simulink model "PRBS_Para_CCPIDSim"  (R2015a)
settings: Solver=ode5  StartTime=0.0  StopTime=10  FixedStep=sim_stepSize
undefined symbols (not defined in the file or in its folder): sim_ccTarget, sim_PIDdGain, sim_PIDiGain, sim_PIDnoise, sim_PIDpGain, sim_PIDsample, sim_Qgain, sim_tracerMax, sim_zoneVolGain
libraries: simulink x8
settings Model: Creator=David  LastModifiedBy=davidveitch
settings SolverCC: NumberNewtonIterations=4  MaxConsecutiveMinStep=auto
settings DataIOCC: LimitDataPoints=off  SaveOutput=off  SignalLogging=off  DSMLogging=off  SaveTime=off  TimeSaveName=d_toutPRBS  OutputSaveName=Conc
settings OptimizationCC: ExpressionDepthLimit=2147483647  SimCompilerOptimization=on
settings DebuggingCC: UnderspecifiedInitializationDetection=Classic  MergeDetectMultiDrivingBlocksExec=none  SolverPrmCheckMsg=warning  MultiTaskRateTransMsg=warning  StateNameClashWarn=warning
settings ModelReferenceCC: UpdateModelReferenceTargets=IfOutOfDate
settings SFSimCC: SFSimEcho=off

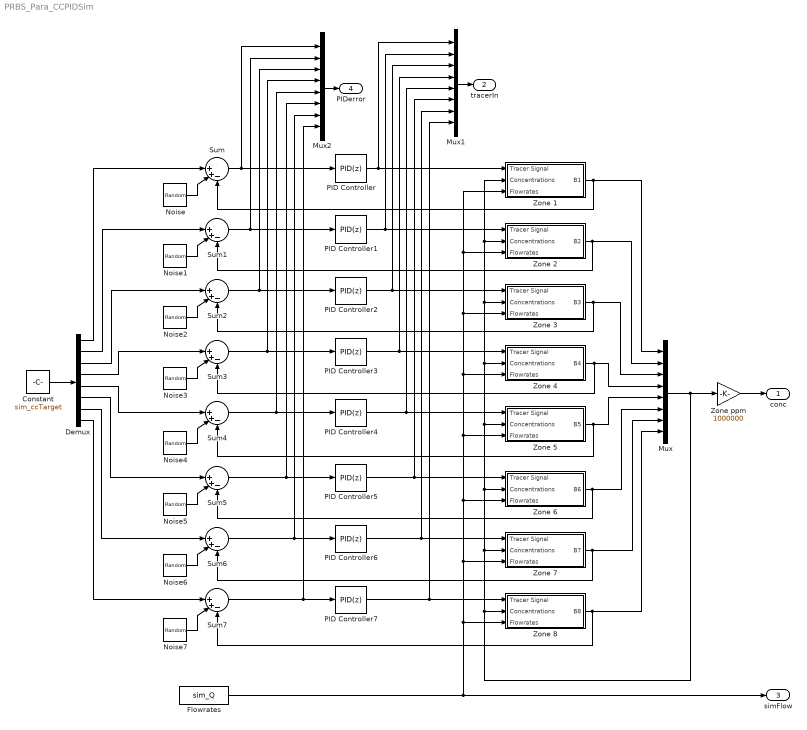
== system PRBS_Para_CCPIDSim ==
  Constant : Constant  Value=sim_ccTarget
  Demux : Demux  Outputs=8
  Flowrates : FromWorkspace  VariableName=sim_Q  SampleTime=0  OutputAfterFinalValue=Holding final value
  Mux : Mux  Inputs=8
  Mux1 : Mux  Inputs=8
  Mux2 : Mux  Inputs=8
  Noise : RandomNumber  Variance=sim_PIDnoise  Seed=100  SampleTime=sim_PIDsample
  Noise1 : RandomNumber  Variance=sim_PIDnoise  Seed=200  SampleTime=sim_PIDsample
  Noise2 : RandomNumber  Variance=sim_PIDnoise  Seed=300  SampleTime=sim_PIDsample
  Noise3 : RandomNumber  Variance=sim_PIDnoise  Seed=400  SampleTime=sim_PIDsample
  Noise4 : RandomNumber  Variance=sim_PIDnoise  Seed=500  SampleTime=sim_PIDsample
  Noise5 : RandomNumber  Variance=sim_PIDnoise  Seed=600  SampleTime=sim_PIDsample
  Noise6 : RandomNumber  Variance=sim_PIDnoise  Seed=700  SampleTime=sim_PIDsample
  Noise7 : RandomNumber  Variance=sim_PIDnoise  Seed=800  SampleTime=sim_PIDsample
  PID Controller{,1..7} (8 alike) : simulink/Continuous/PID Controller  Controller=PID  TimeDomain=Discrete-time  SampleTime=sim_PIDsample  IntegratorMethod=Forward Euler  FilterMethod=Forward Euler  Form=Parallel  UseFilter=on  ControllerParametersSource=internal  P=sim_PIDpGain  I=sim_PIDiGain  D=sim_PIDdGain  N=100  InitialConditionSource=internal  InitialConditionForIntegrator=0  InitialConditionForFilter=0  ExternalReset=none  LimitOutput=on  UpperSaturationLimit=sim_tracerMax  LowerSaturationLimit=0  LinearizeAsGain=on  AntiWindupMode=none  Kb=1  TrackingMode=off  Kt=1  PParamMin=[]  PParamMax=[]  IParamMin=[]  IParamMax=[]  DParamMin=[]  DParamMax=[]  NParamMin=[]  NParamMax=[]  KbParamMin=[]  KbParamMax=[]  KtParamMin=[]  KtParamMax=[]  POutMin=[]  POutMax=[]  IOutMin=[]  IOutMax=[]  DOutMin=[]  DOutMax=[]  NOutMin=[]  NOutMax=[]  KbOutMin=[]  KbOutMax=[]  KtOutMin=[]  KtOutMax=[]  IntegratorOutMin=[]  IntegratorOutMax=[]  FilterOutMin=[]  FilterOutMax=[]  SumOutMin=[]  SumOutMax=[]  SumI1OutMin=[]  SumI1OutMax=[]  SumI2OutMin=[]  SumI2OutMax=[]  SumI3OutMin=[]  SumI3OutMax=[]  SumDOutMin=[]  SumDOutMax=[]  SaturationOutMin=[]  SaturationOutMax=[]  IntegratorContinuousStateAttributes=''  IntegratorStateMustResolveToSignalObject=off  IntegratorRTWStateStorageClass=Auto  FilterContinuousStateAttributes=''  FilterStateMustResolveToSignalObject=off  FilterRTWStateStorageClass=Auto  DifferentiatorICPrevScaledInput=0  DifferentiatorOutMin=[]  DifferentiatorOutMax=[]
  Sum{,1..7} (8 alike) : Sum  Inputs=||++-
  Zone ppm : Gain  Gain=1000000
  Zone 1 : Subsystem
  Zone 2 : Subsystem
  Zone 3 : Subsystem
  Zone 4 : Subsystem
  Zone 5 : Subsystem
  Zone 6 : Subsystem
  Zone 7 : Subsystem
  Zone 8 : Subsystem
  conc : Outport
  tracerIn : Outport  Port=2
  simFlow : Outport  Port=3
  PIDerror : Outport  Port=4
  wires:
  Zone 2/1(B2) -> Sum1/3, Mux/2
  Mux/1 -> Zone ppm/1, Zone 8/2(Concentrations), Zone 7/2(Concentrations), Zone 6/2(Concentrations), Zone 5/2(Concentrations), Zone 4/2(Concentrations), Zone 1/2(Concentrations), Zone 2/2(Concentrations), Zone 3/2(Concentrations)
  Zone ppm/1 -> conc/1
  Flowrates/1 -> simFlow/1, Zone 8/3(Flowrates), Zone 7/3(Flowrates), Zone 6/3(Flowrates), Zone 1/3(Flowrates), Zone 2/3(Flowrates), Zone 3/3(Flowrates), Zone 4/3(Flowrates), Zone 5/3(Flowrates)
  Zone 4/1(B4) -> Sum3/3, Mux/4
  Zone 5/1(B5) -> Sum4/3, Mux/5
  Zone 6/1(B6) -> Sum5/3, Mux/6
  Zone 7/1(B7) -> Sum6/3, Mux/7
  Zone 8/1(B8) -> Sum7/3, Mux/8
  Zone 1/1(B1) -> Sum/3, Mux/1
  PID Controller/1 -> Mux1/1, Zone 1/1(Tracer Signal)
  PID Controller1/1 -> Mux1/2, Zone 2/1(Tracer Signal)
  PID Controller2/1 -> Mux1/3, Zone 3/1(Tracer Signal)
  PID Controller3/1 -> Mux1/4, Zone 4/1(Tracer Signal)
  PID Controller4/1 -> Mux1/5, Zone 5/1(Tracer Signal)
  PID Controller5/1 -> Mux1/6, Zone 6/1(Tracer Signal)
  PID Controller6/1 -> Mux1/7, Zone 7/1(Tracer Signal)
  PID Controller7/1 -> Mux1/8, Zone 8/1(Tracer Signal)
  Constant/1 -> Demux/1
  Demux/1 -> Sum/1
  Demux/2 -> Sum1/1
  Demux/3 -> Sum2/1
  Demux/4 -> Sum3/1
  Demux/5 -> Sum4/1
  Demux/6 -> Sum5/1
  Demux/7 -> Sum6/1
  Demux/8 -> Sum7/1
  Mux1/1 -> tracerIn/1
  Sum/1 -> PID Controller/1, Mux2/1
  Sum1/1 -> Mux2/2, PID Controller1/1
  Sum2/1 -> Mux2/3, PID Controller2/1
  Sum3/1 -> Mux2/4, PID Controller3/1
  Sum4/1 -> Mux2/5, PID Controller4/1
  Sum5/1 -> Mux2/6, PID Controller5/1
  Sum6/1 -> Mux2/7, PID Controller6/1
  Sum7/1 -> Mux2/8, PID Controller7/1
  Zone 3/1(B3) -> Sum2/3, Mux/3
  Noise/1 -> Sum/2
  Noise1/1 -> Sum1/2
  Noise2/1 -> Sum2/2
  Mux2/1 -> PIDerror/1
  Noise7/1 -> Sum7/2
  Noise6/1 -> Sum6/2
  Noise5/1 -> Sum5/2
  Noise4/1 -> Sum4/2
  Noise3/1 -> Sum3/2

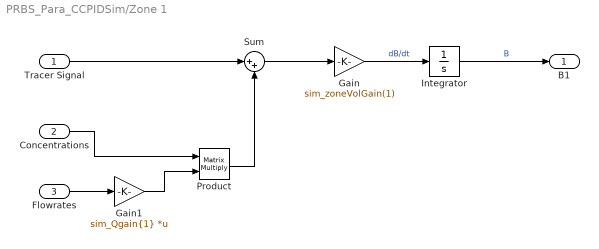
== system PRBS_Para_CCPIDSim/Zone 1 ==
  Tracer Signal : Inport
  Concentrations : Inport  Port=2
  Flowrates : Inport  Port=3
  Gain : Gain  Gain=sim_zoneVolGain(1)
  Gain1 : Gain  Gain=sim_Qgain{1}  Multiplication=Matrix(K*u)
  Integrator : Integrator
  Product : Product  Multiplication=Matrix(*)  RndMeth=Zero
  Sum : Sum  Inputs=|++
  B1 : Outport
  wires:
  Sum/1 -> Gain/1
  Gain/1 -> Integrator/1  "dB/dt"
  Integrator/1 -> B1/1  "B"
  Concentrations/1 -> Product/1
  Product/1 -> Sum/2
  Tracer Signal/1 -> Sum/1
  Flowrates/1 -> Gain1/1
  Gain1/1 -> Product/2

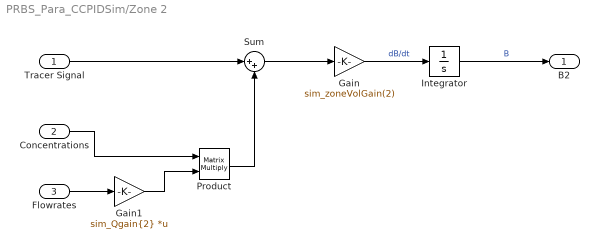
== system PRBS_Para_CCPIDSim/Zone 2 ==
  Tracer Signal : Inport
  Concentrations : Inport  Port=2
  Flowrates : Inport  Port=3
  Gain : Gain  Gain=sim_zoneVolGain(2)
  Gain1 : Gain  Gain=sim_Qgain{2}  Multiplication=Matrix(K*u)
  Integrator : Integrator
  Product : Product  Multiplication=Matrix(*)  RndMeth=Zero
  Sum : Sum  Inputs=|++
  B2 : Outport
  wires:
  Sum/1 -> Gain/1
  Gain/1 -> Integrator/1  "dB/dt"
  Integrator/1 -> B2/1  "B"
  Concentrations/1 -> Product/1
  Product/1 -> Sum/2
  Tracer Signal/1 -> Sum/1
  Flowrates/1 -> Gain1/1
  Gain1/1 -> Product/2

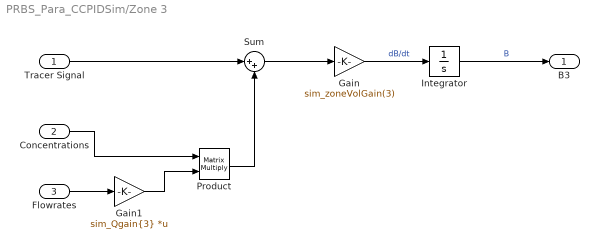
== system PRBS_Para_CCPIDSim/Zone 3 ==
  Tracer Signal : Inport
  Concentrations : Inport  Port=2
  Flowrates : Inport  Port=3
  Gain : Gain  Gain=sim_zoneVolGain(3)
  Gain1 : Gain  Gain=sim_Qgain{3}  Multiplication=Matrix(K*u)
  Integrator : Integrator
  Product : Product  Multiplication=Matrix(*)  RndMeth=Zero
  Sum : Sum  Inputs=|++
  B3 : Outport
  wires:
  Sum/1 -> Gain/1
  Gain/1 -> Integrator/1  "dB/dt"
  Integrator/1 -> B3/1  "B"
  Concentrations/1 -> Product/1
  Product/1 -> Sum/2
  Tracer Signal/1 -> Sum/1
  Flowrates/1 -> Gain1/1
  Gain1/1 -> Product/2

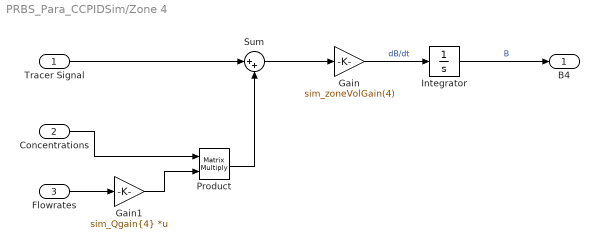
== system PRBS_Para_CCPIDSim/Zone 4 ==
  Tracer Signal : Inport
  Concentrations : Inport  Port=2
  Flowrates : Inport  Port=3
  Gain : Gain  Gain=sim_zoneVolGain(4)
  Gain1 : Gain  Gain=sim_Qgain{4}  Multiplication=Matrix(K*u)
  Integrator : Integrator
  Product : Product  Multiplication=Matrix(*)  RndMeth=Zero
  Sum : Sum  Inputs=|++
  B4 : Outport
  wires:
  Sum/1 -> Gain/1
  Gain/1 -> Integrator/1  "dB/dt"
  Integrator/1 -> B4/1  "B"
  Concentrations/1 -> Product/1
  Product/1 -> Sum/2
  Tracer Signal/1 -> Sum/1
  Flowrates/1 -> Gain1/1
  Gain1/1 -> Product/2

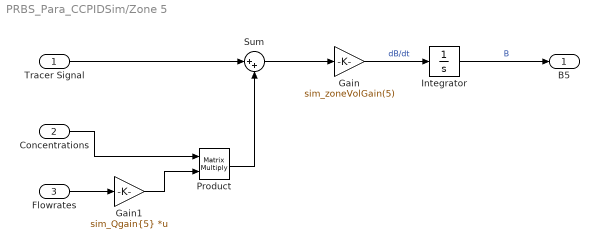
== system PRBS_Para_CCPIDSim/Zone 5 ==
  Tracer Signal : Inport
  Concentrations : Inport  Port=2
  Flowrates : Inport  Port=3
  Gain : Gain  Gain=sim_zoneVolGain(5)
  Gain1 : Gain  Gain=sim_Qgain{5}  Multiplication=Matrix(K*u)
  Integrator : Integrator
  Product : Product  Multiplication=Matrix(*)  RndMeth=Zero
  Sum : Sum  Inputs=|++
  B5 : Outport
  wires:
  Sum/1 -> Gain/1
  Gain/1 -> Integrator/1  "dB/dt"
  Integrator/1 -> B5/1  "B"
  Concentrations/1 -> Product/1
  Product/1 -> Sum/2
  Tracer Signal/1 -> Sum/1
  Flowrates/1 -> Gain1/1
  Gain1/1 -> Product/2

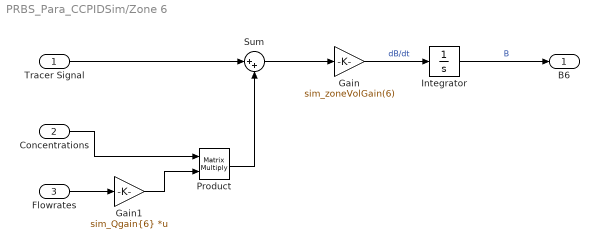
== system PRBS_Para_CCPIDSim/Zone 6 ==
  Tracer Signal : Inport
  Concentrations : Inport  Port=2
  Flowrates : Inport  Port=3
  Gain : Gain  Gain=sim_zoneVolGain(6)
  Gain1 : Gain  Gain=sim_Qgain{6}  Multiplication=Matrix(K*u)
  Integrator : Integrator
  Product : Product  Multiplication=Matrix(*)  RndMeth=Zero
  Sum : Sum  Inputs=|++
  B6 : Outport
  wires:
  Sum/1 -> Gain/1
  Gain/1 -> Integrator/1  "dB/dt"
  Integrator/1 -> B6/1  "B"
  Concentrations/1 -> Product/1
  Product/1 -> Sum/2
  Tracer Signal/1 -> Sum/1
  Flowrates/1 -> Gain1/1
  Gain1/1 -> Product/2

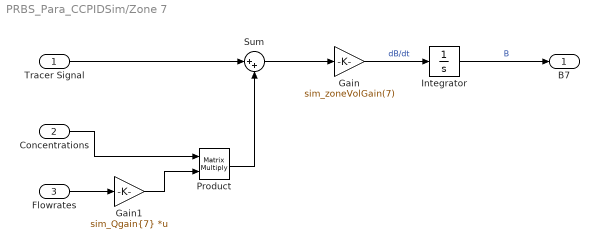
== system PRBS_Para_CCPIDSim/Zone 7 ==
  Tracer Signal : Inport
  Concentrations : Inport  Port=2
  Flowrates : Inport  Port=3
  Gain : Gain  Gain=sim_zoneVolGain(7)
  Gain1 : Gain  Gain=sim_Qgain{7}  Multiplication=Matrix(K*u)
  Integrator : Integrator
  Product : Product  Multiplication=Matrix(*)  RndMeth=Zero
  Sum : Sum  Inputs=|++
  B7 : Outport
  wires:
  Sum/1 -> Gain/1
  Gain/1 -> Integrator/1  "dB/dt"
  Integrator/1 -> B7/1  "B"
  Concentrations/1 -> Product/1
  Product/1 -> Sum/2
  Tracer Signal/1 -> Sum/1
  Flowrates/1 -> Gain1/1
  Gain1/1 -> Product/2

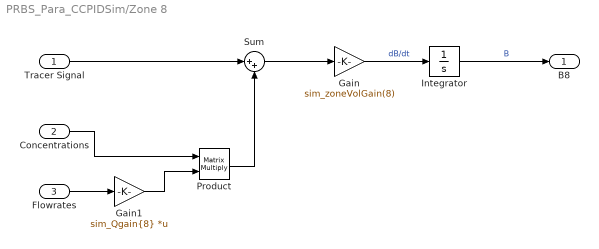
== system PRBS_Para_CCPIDSim/Zone 8 ==
  Tracer Signal : Inport
  Concentrations : Inport  Port=2
  Flowrates : Inport  Port=3
  Gain : Gain  Gain=sim_zoneVolGain(8)
  Gain1 : Gain  Gain=sim_Qgain{8}  Multiplication=Matrix(K*u)
  Integrator : Integrator
  Product : Product  Multiplication=Matrix(*)  RndMeth=Zero
  Sum : Sum  Inputs=|++
  B8 : Outport
  wires:
  Sum/1 -> Gain/1
  Gain/1 -> Integrator/1  "dB/dt"
  Integrator/1 -> B8/1  "B"
  Concentrations/1 -> Product/1
  Product/1 -> Sum/2
  Tracer Signal/1 -> Sum/1
  Flowrates/1 -> Gain1/1
  Gain1/1 -> Product/2
